simulink model "Model_vertical_lqr_2015a"  (R2015a)
settings: Solver=ode4  StartTime=0.0  StopTime=10.0  FixedStep=1e-3  RelTol=1e-3
values from neighbouring files (symbols this model uses):
  a = moment(pwm==0)    [Helicopter_main.m]    (also in Helicopter_main_test.m = moment(pwm==0)/-sin(-0.5223))
  alpha_0 = parameters(3)    [Helicopter_main.m]    (also in Helicopter_main_test.m)
  f_v = parameters(2)    [Helicopter_main.m]    (also in Helicopter_main_test.m)
  I_v = lsqnonlin(cel, I_v, 0,[],options)    [Helicopter_main.m]    (also in Helicopter_main_test.m)
  J_v = parameters(1)    [Helicopter_main.m]    (also in Helicopter_main_test.m)
  K_lqr = lqr(lin_A, lin_B, Q, R, N)    [Helicopter_main.m]    (also in Helicopter_main_test.m)
  L = place(lin_A.', lin_C.', lambda).'    [Helicopter_main.m]    (also in Helicopter_main_test.m)
  lin_A = [0 1 0;     a/J_v*cos(lin_alpha_v-alpha_0) -f_v/J_v polyval(lin_M_V_diff, lin_w_v)/J_v;     0 0 -polyval(lin_U_V_diff, lin_w_v)/I_v]    [Helicopter_main.m]    (also in Helicopter_main_test.m)
  lin_alpha_v = 0    [Helicopter_main.m]    (also in Helicopter_main_test.m)
  lin_B = [0; 0; 1/I_v]    [Helicopter_main.m]    (also in Helicopter_main_test.m)
  lin_C = [1 0 0]    [Helicopter_main.m]    (also in Helicopter_main_test.m)
  lin_u_v = polyval(wsp_U_V, lin_w_v)    [Helicopter_main.m]    (also in Helicopter_main_test.m)
  lin_velocity_v = 0    [Helicopter_main.m]    (also in Helicopter_main_test.m)
  lin_w_v = real(lin_w_v(lin_w_v>-50 & lin_w_v<50 & imag(lin_w_v)==0))    [Helicopter_main.m]    (also in Helicopter_main_test.m = real(lin_w_v(lin_w_v>-350 & lin_w_v<350 & imag(lin_w_v)==0)))
  wsp_M_V = polyfit(v/60, moment, 5)    [Helicopter_main.m]    (also in Helicopter_main_test.m = polyfit(v, moment, 5))
  wsp_U_V = polyfit(pred,PWM,5)    [Helicopter_main.m]    (also in Helicopter_main_test.m)
settings Model: Creator=Student  LastModifiedBy=Student

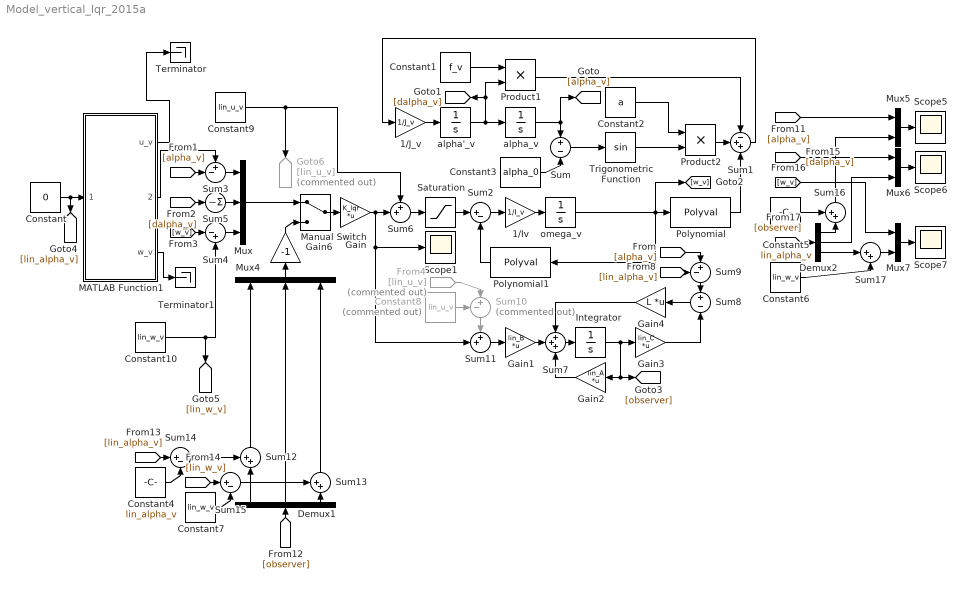
== system Model_vertical_lqr_2015a ==
  1/Iv : Gain  Gain=1/I_v
  1/J_v : Gain  Gain=1/J_v
  Constant : Constant  Value=0
  Constant1 : Constant  Value=f_v
  Constant10 : Constant  Value=lin_w_v
  Constant2 : Constant  Value=a
  Constant3 : Constant  Value=alpha_0
  Constant4 : Constant  Value=lin_alpha_v
  Constant5 : Constant  Value=lin_alpha_v
  Constant6 : Constant  Value=lin_w_v
  Constant7 : Constant  Value=lin_w_v
  Constant8 : Constant  Commented=on  Value=lin_u_v
  Constant9 : Constant  Value=lin_u_v
  Demux1 : Demux  Outputs=3
  Demux2 : Demux  Outputs=3
  From4 : From  Commented=on  GotoTag=lin_u_v
  Gain : Gain  Gain=K_lqr  Multiplication=Matrix(K*u)
  Gain1 : Gain  Gain=lin_B  Multiplication=Matrix(K*u)
  Gain2 : Gain  Gain=lin_A  Multiplication=Matrix(K*u)
  Gain3 : Gain  Gain=lin_C  Multiplication=Matrix(K*u)
  Gain4 : Gain  Gain=L  Multiplication=Matrix(K*u)
  Gain6 : Gain  Gain=-1
  Goto6 : Goto  Commented=on  GotoTag=lin_u_v
  Integrator : Integrator  InitialCondition=[0;0;0]
  MATLAB Function1 : MATLAB Function  TreatAsAtomicUnit=on
  Manual Switch : ManualSwitch
  Mux : Mux  Inputs=3
  Mux4 : Mux  Inputs=3
  Mux5 : Mux  Inputs=2
  Mux6 : Mux  Inputs=2
  Mux7 : Mux  Inputs=2
  Polynomial : Polyval  Coefs=wsp_M_V
  Polynomial1 : Polyval  Coefs=wsp_U_V
  Product1 : Product
  Product2 : Product
  Saturation : Saturate  UpperLimit=1  LowerLimit=-1
  Scope{1,5..7} (4 alike) : Scope
      Scope1 settings: YMin=-0.02014  YMax=0.06521
      Scope5 settings: YMin=-0.03322  YMax=0.12013
      Scope6 settings: YMin=-0.06773  YMax=0.05947  SaveName=ScopeData2
      Scope7 settings: YMin=171.46242  YMax=188.98603  SaveName=ScopeData3
  Sum : Sum  Inputs=+|-
  Sum1 : Sum  Inputs=-++
  Sum10 : Sum  Commented=on  Inputs=-+|
  Sum{6,11..13,16} (5 alike) : Sum  Inputs=++|
  Sum14 : Sum  Inputs=|+-
  Sum15 : Sum  Inputs=|+-
  Sum17 : Sum  Inputs=|++
  Sum2 : Sum  Inputs=|+-
  Sum3 : Sum  Inputs=+-|
  Sum4 : Sum  Inputs=|-+
  Sum5 : Sum  Inputs=|-|
  Sum7 : Sum  Inputs=+++
  Sum8 : Sum  Inputs=+|-
  Sum9 : Sum  Inputs=-+|
  Terminator : Terminator
  Terminator1 : Terminator
  Trigonometric Function : Trigonometry
  alpha'_v : Integrator  InitialCondition=lin_velocity_v
  alpha_v : Integrator  InitialCondition=lin_alpha_v+0.1
  omega_v : Integrator  InitialCondition=lin_w_v
  wires:
  omega_v/1 -> [w_v], Polynomial1/1, Polynomial/1
  Product2/1 -> Sum1/2
  Sum2/1 -> 1/Iv/1
  Sum/1 -> Trigonometric Function/1
  Constant3/1 -> Sum/2
  Constant1/1 -> Product1/1
  alpha_v/1 -> [alpha_v], Sum/1
  Constant2/1 -> Product2/1
  Polynomial/1 -> Sum1/3
  Sum1/1 -> 1/J_v/1
  Product1/1 -> Sum1/1
  1/J_v/1 -> alpha'_v/1
  alpha'_v/1 -> [dalpha_v], Product1/2, alpha_v/1
  Trigonometric Function/1 -> Product2/2
  Polynomial1/1 -> Sum2/2
  1/Iv/1 -> omega_v/1
  [alpha_v] -> Sum9/2
  [alpha_v] -> Sum3/2
  Sum3/1 -> Mux/1
  MATLAB Function1/2(alpha_v) -> Sum3/1
  Sum4/1 -> Mux/3
  [w_v] -> Sum4/1
  [dalpha_v] -> Sum5/1
  Sum5/1 -> Mux/2
  Sum6/1 -> Saturation/1
  Saturation/1 -> Sum2/1
  Gain1/1 -> Sum7/2
  Sum7/1 -> Integrator/1
  Gain2/1 -> Sum7/3
  Integrator/1 -> Gain3/1, [observer], Gain2/1
  Gain3/1 -> Sum8/2
  Sum8/1 -> Gain4/1
  Gain4/1 -> Sum7/1
  Gain/1 -> Sum11/2, Scope1/1, Sum6/2
  Constant/1 -> MATLAB Function1/1(alpha_vin), [lin_alpha_v]
  Sum9/1 -> Sum8/1
  [lin_alpha_v] -> Sum9/1
  Manual Switch/1 -> Gain/1
  Mux/1 -> Manual Switch/1
  Gain6/1 -> Manual Switch/2
  Sum13/1 -> Mux4/3
  Mux4/1 -> Gain6/1
  Sum12/1 -> Mux4/1
  [observer] -> Demux1/1
  Demux1/1 -> Sum12/2
  Demux1/2 -> Mux4/2
  Demux1/3 -> Sum13/2
  Sum14/1 -> Sum12/1
  Sum15/1 -> Sum13/1
  Constant7/1 -> Sum15/2
  [lin_alpha_v] -> Sum14/1
  [lin_w_v] -> Sum15/1
  Constant4/1 -> Sum14/2
  [dalpha_v] -> Mux6/1
  Sum16/1 -> Mux5/2
  Mux7/1 -> Scope7/1
  Demux2/3 -> Sum17/1
  Mux5/1 -> Scope5/1
  Demux2/1 -> Sum16/2
  Sum17/1 -> Mux7/2
  Mux6/1 -> Scope6/1
  [observer] -> Demux2/1
  Constant6/1 -> Sum17/2
  [w_v] -> Mux7/1
  Demux2/2 -> Mux6/2
  Constant5/1 -> Sum16/1
  [alpha_v] -> Mux5/1
  Sum11/1 -> Gain1/1
  Sum10/1 -> Sum11/1
  From4/1 -> Sum10/2
  Constant8/1 -> Sum10/1
  Constant9/1 -> Goto6/1, Sum6/1
  MATLAB Function1/1(u_v) -> Terminator/1
  Constant10/1 -> Sum4/2, [lin_w_v]
  MATLAB Function1/3(w_v) -> Terminator1/1

== matlab function Model_vertical_lqr_2015a/MATLAB Function1 ==
  data: u_v output double size=1 [0..1]; alpha_vin input; alpha_v output; w_v output double size=1
function [u_v, alpha_v, w_v] = Lin(alpha_vin)

const = load('Lin_simulink_test.mat');

w_v = roots(const.wsp_M_V+[zeros(1,length(const.wsp_M_V)-1) const.a*sin(alpha_vin-const.alpha_0)]);
w_v = real(w_v(w_v>-350 & w_v<350 & imag(w_v)==0));
w_v = w_v(1);
u_v = polyval(const.wsp_U_V, w_v);
u_v = u_v(1);
alpha_v = alpha_vin;
